simulink model "mariner_sim"  (R2018b)
settings: Solver=ode1  StartTime=0.0  StopTime=600  FixedStep=0.1  RelTol=1e-3
libraries: neural x408, simulink x2
(part 12 of 22)

== system mariner_sim/Plant/NN Plant mariner (no delta_dot) pre and post processing/Layer 6/Delays 1 ==
  "p{6}" : Inport  PortDimensions=24
      mask Display: e = 0.06;c1 = [120 230 180]/255;c2 = ([120 230 180]+0)/(256+128);c3 = ([120 230 180]+128)/(256+128);patch([0 1 1 0],[0 0 1 1],c1);patch([0 1 1 1-e 1-e 0+e],[0 0 1 1-e 0+e 0+e],c2);patch([0 0 1 1-e 0+e 0+e],[0 1 1 1-e 1-e 0+e],c3);plot([0 1 1 0 0],[0 0 1 1 0]);
  mux : Mux  Inputs=1
      mask Display: e = 0.06;c1 = [120 150 230]/255;c2 = ([120 150 230]+0)/383;c3 = ([120 150 230]+128)/383;patch([0 1 1 0],[0 0 1 1],c1);patch([0 1 1 1-e 1-e 0+e],[0 0 1 1-e 0+e 0+e],c2);patch([0 0 1 1-e 0+e 0+e],[0 1 1 1-e 1-e 0+e],c3);plot([0 1 1 0 0],[0 0 1 1 0]);disp('Mux')
  "pd{6,5}" : Outport
      mask Display: e = 0.06;c1 = [120 230 180]/255;c2 = ([120 230 180]+0)/(256+128);c3 = ([120 230 180]+128)/(256+128);patch([0 1 1 0],[0 0 1 1],c1);patch([0 1 1 1-e 1-e 0+e],[0 0 1 1-e 0+e 0+e],c2);patch([0 0 1 1-e 0+e 0+e],[0 1 1 1-e 1-e 0+e],c3);plot([0 1 1 0 0],[0 0 1 1 0]);
  wires:
  mux/1 -> "pd{6,5}"/1
  "p{6}"/1 -> mux/1

== system mariner_sim/Plant/NN Plant mariner (no delta_dot) pre and post processing/Layer 6/LW{6,5} ==
  "ad{6,5}" : Inport  PortDimensions=24
      mask Display: e = 0.06;c1 = [120 230 180]/255;c2 = ([120 230 180]+0)/(256+128);c3 = ([120 230 180]+128)/(256+128);patch([0 1 1 0],[0 0 1 1],c1);patch([0 1 1 1-e 1-e 0+e],[0 0 1 1-e 0+e 0+e],c2);patch([0 0 1 1-e 0+e 0+e],[0 1 1 1-e 1-e 0+e],c3);plot([0 1 1 0 0],[0 0 1 1 0]);
  "IW{6,5}(1,:)'" : Constant  Value=[-0.1984734159113137608176913317947764880955219268798828125;0.341861037683038826440196089606615714728832244873046875;0.3514792256180998553105609971680678427219390869140625;0.0708036460294599045983687801708583720028400421142578125;-0.2060005329274126051330995323951356112957000732421875;-0.28458774915436857444461793420487083494663238525390625;0.34526917716851002193578779042582027614116668701171875;0.252498381251613224218743880555848591029644012451171875;0.382796941171386462254844218477956019341945648193359375;0.1069087646510679390221554285744787193834781646728515625;0.265337792837605002116418972946121357381343841552734375;-0.0036982135335794073284498839626621702336706221103668212890625;0.097003491573064704045492590012145228683948516845703125;0.337797072626230543423986318884999491274356842041015625;-0.2407305535513760974541952464278438128530979156494140625;0.032264868090931257682552057985958526842296123504638671875;-0.09944305951370562002278319368997472338378429412841796875;-0.0237766981619511319490101186602259986102581024169921875;-0.368802813456096723054855601731105707585811614990234375;-0.0342788950269383996261041147590731270611286163330078125;-0.3817990555449328748949255896150134503841400146484375;-0.337620208706587543456834055177750997245311737060546875;0.2156801313526628127714701577133382670581340789794921875;0.487288760457548264515281744024832732975482940673828125]
      mask Display: e = 0.06;c1 = [120 150 230]/255;c2 = ([120 150 230]+0)/383;c3 = ([120 150 230]+128)/383;patch([0 1 1 0],[0 0 1 1],c1);patch([0 1 1 1-e 1-e 0+e],[0 0 1 1-e 0+e 0+e],c2);patch([0 0 1 1-e 0+e 0+e],[0 1 1 1-e 1-e 0+e],c3);plot([0 1 1 0 0],[0 0 1 1 0]);disp('weights');
  "IW{6,5}(2,:)'" : Constant  Value=[-0.09751875485376855501318260621701483614742755889892578125;0.01035142127946475643085477713611908257007598876953125;-0.0633120424566557538081923439676756970584392547607421875;0.1178993640669732390069412986122188158333301544189453125;0.09018636110401789807156092138029634952545166015625;-0.2332660662459413725144941054168157279491424560546875;0.06980453513620508976256218147682375274598598480224609375;0.1317458131781703845053499435380217619240283966064453125;-0.1974794491107817184794015474835759960114955902099609375;0.045960960379689101695799280378196272067725658416748046875;-0.0286857227069632104987650933480836101807653903961181640625;0.031652413341904737931198354772277525626122951507568359375;-0.1798477845368142979953773874512990005314350128173828125;0.113930975779332255282128016915521584451198577880859375;-0.1329135904041280069609598513125092722475528717041015625;0.1710109273118207984243355213038739748299121856689453125;-0.395146018496356277172054660695721395313739776611328125;0.0157313605677542878158448047543060965836048126220703125;-0.2089047495222683681337372263442375697195529937744140625;-0.012458230094540577448380958003326668404042720794677734375;0.1814413847518826783389300771887064911425113677978515625;0.16440010903084878446378525040927343070507049560546875;-0.0299410897703677979231340344767886563204228878021240234375;-0.291647538202252476491338484265725128352642059326171875]
      mask Display: e = 0.06;c1 = [120 150 230]/255;c2 = ([120 150 230]+0)/383;c3 = ([120 150 230]+128)/383;patch([0 1 1 0],[0 0 1 1],c1);patch([0 1 1 1-e 1-e 0+e],[0 0 1 1-e 0+e 0+e],c2);patch([0 0 1 1-e 0+e 0+e],[0 1 1 1-e 1-e 0+e],c3);plot([0 1 1 0 0],[0 0 1 1 0]);disp('weights');
  "IW{6,5}(3,:)'" : Constant  Value=[0.107561595046206937009714010855532251298427581787109375;0.11473176770232372534419340581735013984143733978271484375;0.09835083216250127546853576632202020846307277679443359375;-0.1101936730172489442569627726697945035994052886962890625;0.01956165002644803807552165153538226149976253509521484375;-0.00138938835503763674118771209720080150873400270938873291015625;0.229539681556379993043748299896833486855030059814453125;-0.02781216225646444828445424946039565838873386383056640625;-0.066868172082727606042595880353474058210849761962890625;-0.06345845663674787306973712475155480206012725830078125;-0.1061321176180718139914205266904900781810283660888671875;0.166181117806918077217659401867422275245189666748046875;0.049588349948201472516817744917716481722891330718994140625;0.038948608670263007436318503096117638051509857177734375;0.013791532259307952290594556643554824404418468475341796875;0.09946765208005929614909490510399336926639080047607421875;-0.11249367046046228335587358060365659184753894805908203125;-0.012219618567312066914620771740374038927257061004638671875;-0.16240728937219872651809282615431584417819976806640625;0.023389458205694983738975878395649488084018230438232421875;0.26389662063826035964808625067234970629215240478515625;0.159727556975424678231689767926582135260105133056640625;0.0754751463558475388371249437113874591886997222900390625;-0.17697164411906440850685839905054308474063873291015625]
      mask Display: e = 0.06;c1 = [120 150 230]/255;c2 = ([120 150 230]+0)/383;c3 = ([120 150 230]+128)/383;patch([0 1 1 0],[0 0 1 1],c1);patch([0 1 1 1-e 1-e 0+e],[0 0 1 1-e 0+e 0+e],c2);patch([0 0 1 1-e 0+e 0+e],[0 1 1 1-e 1-e 0+e],c3);plot([0 1 1 0 0],[0 0 1 1 0]);disp('weights');
  "IW{6,5}(4,:)'" : Constant  Value=[-0.024147515529926721900011443722178228199481964111328125;-0.115126686689287882625620795806753449141979217529296875;-0.13186707320813206845144804901792667806148529052734375;-0.045328318661101707487404155472177080810070037841796875;-0.2033729362155631548159107069295714609324932098388671875;0.07246896249946392642993231447690050117671489715576171875;-0.2179812681494835702178392011774121783673763275146484375;0.297405231087761456887363920031930319964885711669921875;0.032114410553897569655656951681521604768931865692138671875;0.04623473238628690584750557945881155319511890411376953125;-0.03509861948767252493031065796458278782665729522705078125;0.364105084360460573567053188526188023388385772705078125;-0.148060441730926084513697560396394692361354827880859375;0.3020276997199451418651960921124555170536041259765625;-0.1543730986813571515181564564045402221381664276123046875;0.10453222125549561927204678113412228412926197052001953125;0.0682407958586081220264674129794002510607242584228515625;0.03498961749381442054573909672399167902767658233642578125;-0.07624817135712991245100056403316557407379150390625;-0.010644929451439501255638475640807882882654666900634765625;-0.132186238467594530110460482319467701017856597900390625;0.320961225121417170758064685287536121904850006103515625;0.287195938470433009825910630752332508563995361328125;-0.112442449440882941136266026660450734198093414306640625]
      mask Display: e = 0.06;c1 = [120 150 230]/255;c2 = ([120 150 230]+0)/383;c3 = ([120 150 230]+128)/383;patch([0 1 1 0],[0 0 1 1],c1);patch([0 1 1 1-e 1-e 0+e],[0 0 1 1-e 0+e 0+e],c2);patch([0 0 1 1-e 0+e 0+e],[0 1 1 1-e 1-e 0+e],c3);plot([0 1 1 0 0],[0 0 1 1 0]);disp('weights');
  "IW{6,5}(5,:)'" : Constant  Value=[0.0265249665311167066861219865359089453704655170440673828125;-0.06515276408474486580235662813720409758388996124267578125;0.11698791214771177282560898902374901808798313140869140625;0.058168059701191376920093034641467966139316558837890625;0.033920652373470742968475377665527048520743846893310546875;-0.09949568443026289565889186405911459587514400482177734375;0.06389822026648651898117492464734823442995548248291015625;-0.007795113443349485811417753922114570741541683673858642578125;0.1501300297768707603385252014049910940229892730712890625;0.07298433793207532993552177913443301804363727569580078125;-0.045143535446797673771346381954572279937565326690673828125;0.013778305668310057707781624003473552875220775604248046875;-0.06351331399283564882463082312824553810060024261474609375;0.1773286164884585180967491169212735258042812347412109375;0.124255763394060136928231941055855713784694671630859375;0.0106476607074032399158358686008796212263405323028564453125;-0.10051592027657681172048143025676836259663105010986328125;0.040941784790665514126573043540702201426029205322265625;0.2495698746379401422590404990842216648161411285400390625;-0.057979253144741782488580383869702927768230438232421875;0.1432954740414220384803201113754766993224620819091796875;-0.12450573687530662458922137147965258918702602386474609375;0.0273682257852485462390479398209208738990128040313720703125;-0.0272394570136111520419763820655134622938930988311767578125]
      mask Display: e = 0.06;c1 = [120 150 230]/255;c2 = ([120 150 230]+0)/383;c3 = ([120 150 230]+128)/383;patch([0 1 1 0],[0 0 1 1],c1);patch([0 1 1 1-e 1-e 0+e],[0 0 1 1-e 0+e 0+e],c2);patch([0 0 1 1-e 0+e 0+e],[0 1 1 1-e 1-e 0+e],c3);plot([0 1 1 0 0],[0 0 1 1 0]);disp('weights');
  "IW{6,5}(6,:)'" : Constant  Value=[-0.2004844681319393473462042720711906440556049346923828125;0.128833455962125864591172330619883723556995391845703125;0.098423568038649877909307406298466958105564117431640625;0.144999619851042316209799309945083223283290863037109375;-0.132357170363239740051852777469321154057979583740234375;0.11375979409283366872163156813257955946028232574462890625;0.06915188401280171481833036750686005689203739166259765625;0.022246094065410081108691286999601288698613643646240234375;-0.11652469676553868505042288461481803096830844879150390625;0.05101664210318289371937083842567517422139644622802734375;-0.05340684599345039973439241975938784889876842498779296875;-0.07022774922811247932941114413551986217498779296875;-0.06459404659984717411713717183374683372676372528076171875;-0.09188557076911878229719121691232430748641490936279296875;-0.0280421329569854015095753396735744900070130825042724609375;-0.131619071904788553784015903147519566118717193603515625;-0.0087761563220312942268375167031990713439881801605224609375;-0.1562829536434182375881363213920849375426769256591796875;0.058614224683764086509807356151213753037154674530029296875;-0.04989826144070728941581904791746637783944606781005859375;-0.06141680902619907345130201292704441584646701812744140625;-0.0230427291839343344193036244860195438377559185028076171875;0.1430616608072586004585247110298951156437397003173828125;-0.10004233012849218786843863426838652230799198150634765625]
      mask Display: e = 0.06;c1 = [120 150 230]/255;c2 = ([120 150 230]+0)/383;c3 = ([120 150 230]+128)/383;patch([0 1 1 0],[0 0 1 1],c1);patch([0 1 1 1-e 1-e 0+e],[0 0 1 1-e 0+e 0+e],c2);patch([0 0 1 1-e 0+e 0+e],[0 1 1 1-e 1-e 0+e],c3);plot([0 1 1 0 0],[0 0 1 1 0]);disp('weights');
  Mux : Mux  Inputs=6
      mask Display: e = 0.06;c1 = [120 150 230]/255;c2 = ([120 150 230]+0)/383;c3 = ([120 150 230]+128)/383;patch([0 1 1 0],[0 0 1 1],c1);patch([0 1 1 1-e 1-e 0+e],[0 0 1 1-e 0+e 0+e],c2);patch([0 0 1 1-e 0+e 0+e],[0 1 1 1-e 1-e 0+e],c3);plot([0 1 1 0 0],[0 0 1 1 0]);disp('Mux');
  dotprod{1..6} (6 alike) : neural/Weight Functions/dotprod
  "lz{6,5}" : Outport
      mask Display: e = 0.06;c1 = [120 230 180]/255;c2 = ([120 230 180]+0)/(256+128);c3 = ([120 230 180]+128)/(256+128);patch([0 1 1 0],[0 0 1 1],c1);patch([0 1 1 1-e 1-e 0+e],[0 0 1 1-e 0+e 0+e],c2);patch([0 0 1 1-e 0+e 0+e],[0 1 1 1-e 1-e 0+e],c3);plot([0 1 1 0 0],[0 0 1 1 0]);
  wires:
  Mux/1 -> "lz{6,5}"/1
  dotprod6/1 -> Mux/6
  "IW{6,5}(6,:)'"/1 -> dotprod6/1
  dotprod5/1 -> Mux/5
  "IW{6,5}(5,:)'"/1 -> dotprod5/1
  dotprod4/1 -> Mux/4
  "IW{6,5}(4,:)'"/1 -> dotprod4/1
  dotprod3/1 -> Mux/3
  "IW{6,5}(3,:)'"/1 -> dotprod3/1
  dotprod2/1 -> Mux/2
  "IW{6,5}(2,:)'"/1 -> dotprod2/1
  dotprod1/1 -> Mux/1
  "ad{6,5}"/1 -> dotprod6/2, dotprod5/2, dotprod4/2, dotprod3/2, dotprod2/2, dotprod1/2
  "IW{6,5}(1,:)'"/1 -> dotprod1/1

== system mariner_sim/Plant/NN plant mariner (No delta_dot)/Layer 1/Delays 1 ==
  "p{1}" : Inport  PortDimensions=8
      mask Display: e = 0.06;c1 = [120 230 180]/255;c2 = ([120 230 180]+0)/(256+128);c3 = ([120 230 180]+128)/(256+128);patch([0 1 1 0],[0 0 1 1],c1);patch([0 1 1 1-e 1-e 0+e],[0 0 1 1-e 0+e 0+e],c2);patch([0 0 1 1-e 0+e 0+e],[0 1 1 1-e 1-e 0+e],c3);plot([0 1 1 0 0],[0 0 1 1 0]);
  mux : Mux  Inputs=1
      mask Display: e = 0.06;c1 = [120 150 230]/255;c2 = ([120 150 230]+0)/383;c3 = ([120 150 230]+128)/383;patch([0 1 1 0],[0 0 1 1],c1);patch([0 1 1 1-e 1-e 0+e],[0 0 1 1-e 0+e 0+e],c2);patch([0 0 1 1-e 0+e 0+e],[0 1 1 1-e 1-e 0+e],c3);plot([0 1 1 0 0],[0 0 1 1 0]);disp('Mux')
  "pd{1,1}" : Outport
      mask Display: e = 0.06;c1 = [120 230 180]/255;c2 = ([120 230 180]+0)/(256+128);c3 = ([120 230 180]+128)/(256+128);patch([0 1 1 0],[0 0 1 1],c1);patch([0 1 1 1-e 1-e 0+e],[0 0 1 1-e 0+e 0+e],c2);patch([0 0 1 1-e 0+e 0+e],[0 1 1 1-e 1-e 0+e],c3);plot([0 1 1 0 0],[0 0 1 1 0]);
  wires:
  mux/1 -> "pd{1,1}"/1
  "p{1}"/1 -> mux/1

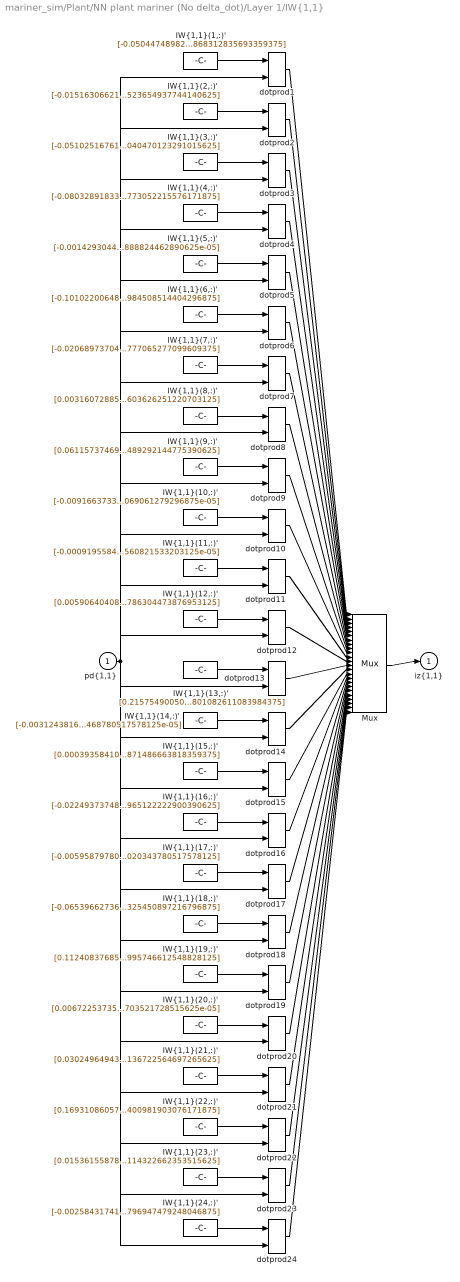
== system mariner_sim/Plant/NN plant mariner (No delta_dot)/Layer 1/IW{1,1} ==
  "pd{1,1}" : Inport  PortDimensions=8
      mask Display: e = 0.06;c1 = [120 230 180]/255;c2 = ([120 230 180]+0)/(256+128);c3 = ([120 230 180]+128)/(256+128);patch([0 1 1 0],[0 0 1 1],c1);patch([0 1 1 1-e 1-e 0+e],[0 0 1 1-e 0+e 0+e],c2);patch([0 0 1 1-e 0+e 0+e],[0 1 1 1-e 1-e 0+e],c3);plot([0 1 1 0 0],[0 0 1 1 0]);
  "IW{1,1}(1,:)'" : Constant  Value=[-0.050447489823092876715104893037278088741004467010498046875;-0.1453020904126429702074574379366822540760040283203125;0.1360442313365746447306747768379864282906055450439453125;0.083616133415922389016117222126922570168972015380859375;0.1859380844177798974836690604206523858010768890380859375;-0.0941200190030648531358536956759053282439708709716796875;-0.09836132576834526186626561639059218578040599822998046875;-0.0022978521690476898763078050791364148608408868312835693359375]
      mask Display: e = 0.06;c1 = [120 150 230]/255;c2 = ([120 150 230]+0)/383;c3 = ([120 150 230]+128)/383;patch([0 1 1 0],[0 0 1 1],c1);patch([0 1 1 1-e 1-e 0+e],[0 0 1 1-e 0+e 0+e],c2);patch([0 0 1 1-e 0+e 0+e],[0 1 1 1-e 1-e 0+e],c3);plot([0 1 1 0 0],[0 0 1 1 0]);disp('Weights');
  "IW{1,1}(10,:)'" : Constant  Value=[-0.00916637331366429268519890882771505857817828655242919921875;-0.0266038197254272502922933796298821107484400272369384765625;0.0179380205035220043063848294195850030519068241119384765625;0.07356487590796183251296014304898562841117382049560546875;0.073478906888268358255089651720481924712657928466796875;-0.0279816931304800974034119320776881068013608455657958984375;0.031718113041040503496947877692946349270641803741455078125;6.7575586318192662200858567000949506109463982284069061279296875e-05]
      mask Display: e = 0.06;c1 = [120 150 230]/255;c2 = ([120 150 230]+0)/383;c3 = ([120 150 230]+128)/383;patch([0 1 1 0],[0 0 1 1],c1);patch([0 1 1 1-e 1-e 0+e],[0 0 1 1-e 0+e 0+e],c2);patch([0 0 1 1-e 0+e 0+e],[0 1 1 1-e 1-e 0+e],c3);plot([0 1 1 0 0],[0 0 1 1 0]);disp('Weights');
  "IW{1,1}(11,:)'" : Constant  Value=[-0.0009195584270885333831591079700729096657596528530120849609375;-0.00444740981314047274797207620622430113144218921661376953125;0.00185387619551044395029004707708963906043209135532379150390625;-2.990664367495710310065719361727332170630688779056072235107421875e-05;0.00051533395249505546502344355275226917001418769359588623046875;-0.004831619154884273480143885848292484297417104244232177734375;-0.00394511335257156058042848911782130016945302486419677734375;5.913357744835549410951369697642121536773629486560821533203125e-05]
      mask Display: e = 0.06;c1 = [120 150 230]/255;c2 = ([120 150 230]+0)/383;c3 = ([120 150 230]+128)/383;patch([0 1 1 0],[0 0 1 1],c1);patch([0 1 1 1-e 1-e 0+e],[0 0 1 1-e 0+e 0+e],c2);patch([0 0 1 1-e 0+e 0+e],[0 1 1 1-e 1-e 0+e],c3);plot([0 1 1 0 0],[0 0 1 1 0]);disp('Weights');
  "IW{1,1}(12,:)'" : Constant  Value=[0.00590640408656031325185242764064241782762110233306884765625;0.00946153844084494412280950115246014320291578769683837890625;0.045269779862591112695735517945649917237460613250732421875;-0.003115516324658056113161563871472026221454143524169921875;-0.0408351532164521469070450621074996888637542724609375;0.0401849319427296791662485020424355752766132354736328125;0.00154371223938102285211382280749603523872792720794677734375;-0.00080467620072569652663052597318937841919250786304473876953125]
      mask Display: e = 0.06;c1 = [120 150 230]/255;c2 = ([120 150 230]+0)/383;c3 = ([120 150 230]+128)/383;patch([0 1 1 0],[0 0 1 1],c1);patch([0 1 1 1-e 1-e 0+e],[0 0 1 1-e 0+e 0+e],c2);patch([0 0 1 1-e 0+e 0+e],[0 1 1 1-e 1-e 0+e],c3);plot([0 1 1 0 0],[0 0 1 1 0]);disp('Weights');
  "IW{1,1}(13,:)'" : Constant  Value=[0.2157549005085194482322918929639854468405246734619140625;-0.21489809351830990724607772790477611124515533447265625;0.0288618450207983497091124291955566150136291980743408203125;-0.237729440761487886835112703920458443462848663330078125;-0.1626972710404361033287301552263670600950717926025390625;0.1747282626319985598950523808525758795440196990966796875;-0.0890875473259058192621040461744996719062328338623046875;-0.002758099109225537436118624867731341510079801082611083984375]
      mask Display: e = 0.06;c1 = [120 150 230]/255;c2 = ([120 150 230]+0)/383;c3 = ([120 150 230]+128)/383;patch([0 1 1 0],[0 0 1 1],c1);patch([0 1 1 1-e 1-e 0+e],[0 0 1 1-e 0+e 0+e],c2);patch([0 0 1 1-e 0+e 0+e],[0 1 1 1-e 1-e 0+e],c3);plot([0 1 1 0 0],[0 0 1 1 0]);disp('Weights');
  "IW{1,1}(14,:)'" : Constant  Value=[-0.0031243816162635413592740807331438190885819494724273681640625;-0.000928296421632138495268204980703785622608847916126251220703125;0.015765539928008949488447143494340707547962665557861328125;0.048519301693036365197286841066670604050159454345703125;0.06761290639592125450985093948474968783557415008544921875;-0.04476563135199958243237716715157148428261280059814453125;0.03100967803026542790600927901323302648961544036865234375;-9.452913233270264612047306673758839679067023098468780517578125e-05]
      mask Display: e = 0.06;c1 = [120 150 230]/255;c2 = ([120 150 230]+0)/383;c3 = ([120 150 230]+128)/383;patch([0 1 1 0],[0 0 1 1],c1);patch([0 1 1 1-e 1-e 0+e],[0 0 1 1-e 0+e 0+e],c2);patch([0 0 1 1-e 0+e 0+e],[0 1 1 1-e 1-e 0+e],c3);plot([0 1 1 0 0],[0 0 1 1 0]);disp('Weights');
  "IW{1,1}(15,:)'" : Constant  Value=[0.0003935841078905092890218020418302558027789928019046783447265625;-0.1219146255765612141264142564978101290762424468994140625;0.126057270212479644033720660445396788418292999267578125;0.26297717154439748110661412283661775290966033935546875;0.04385614172394687593214968046595458872616291046142578125;-0.1216715595383603132351169051617034710943698883056640625;-0.2243991548874049446471445889983442611992359161376953125;-0.00273468434944550663201479068220578483305871486663818359375]
      mask Display: e = 0.06;c1 = [120 150 230]/255;c2 = ([120 150 230]+0)/383;c3 = ([120 150 230]+128)/383;patch([0 1 1 0],[0 0 1 1],c1);patch([0 1 1 1-e 1-e 0+e],[0 0 1 1-e 0+e 0+e],c2);patch([0 0 1 1-e 0+e 0+e],[0 1 1 1-e 1-e 0+e],c3);plot([0 1 1 0 0],[0 0 1 1 0]);disp('Weights');
  "IW{1,1}(16,:)'" : Constant  Value=[-0.022493737485670149689465091569218202494084835052490234375;-0.02601958225636073762654376650971244089305400848388671875;0.0102396778713121604231783834393354482017457485198974609375;-0.00708757931484025986701436039538748445920646190643310546875;-0.00939306055311749099612228519617929123342037200927734375;-0.023126191692564530832942892857317929156124591827392578125;-0.011058591516381617581021856722145457752048969268798828125;0.0003539120631967357225901305017856657286756671965122222900390625]
      mask Display: e = 0.06;c1 = [120 150 230]/255;c2 = ([120 150 230]+0)/383;c3 = ([120 150 230]+128)/383;patch([0 1 1 0],[0 0 1 1],c1);patch([0 1 1 1-e 1-e 0+e],[0 0 1 1-e 0+e 0+e],c2);patch([0 0 1 1-e 0+e 0+e],[0 1 1 1-e 1-e 0+e],c3);plot([0 1 1 0 0],[0 0 1 1 0]);disp('Weights');
  "IW{1,1}(17,:)'" : Constant  Value=[-0.005958797805897233547389735264232513145543634891510009765625;-0.0093973397642727225786973832555304397828876972198486328125;-0.0012376240122008541448550555941210404853336513042449951171875;-0.00065132841794760822605458994161153896129690110683441162109375;-4.5122076628949407748996047740064341269317083060741424560546875e-05;-0.00805713876593570042794478780479039414785802364349365234375;-0.0102162154296771591488468544639545143581926822662353515625;0.0001810033460837132297804874525581908528693020343780517578125]
      mask Display: e = 0.06;c1 = [120 150 230]/255;c2 = ([120 150 230]+0)/383;c3 = ([120 150 230]+128)/383;patch([0 1 1 0],[0 0 1 1],c1);patch([0 1 1 1-e 1-e 0+e],[0 0 1 1-e 0+e 0+e],c2);patch([0 0 1 1-e 0+e 0+e],[0 1 1 1-e 1-e 0+e],c3);plot([0 1 1 0 0],[0 0 1 1 0]);disp('Weights');
  "IW{1,1}(18,:)'" : Constant  Value=[-0.0653966273670904818526850021953578107059001922607421875;-0.0035273106601568355276954402910405406146310269832611083984375;0.12142031588376388240302361509748152457177639007568359375;0.005048567160771975058375371503416317864321172237396240234375;-0.0230617190358675637484875409199958085082471370697021484375;0.12134561262626984701196164451175718568265438079833984375;-0.0821387603606360539032493761624209582805633544921875;-0.002553882405162404001242038020791369490325450897216796875]
      mask Display: e = 0.06;c1 = [120 150 230]/255;c2 = ([120 150 230]+0)/383;c3 = ([120 150 230]+128)/383;patch([0 1 1 0],[0 0 1 1],c1);patch([0 1 1 1-e 1-e 0+e],[0 0 1 1-e 0+e 0+e],c2);patch([0 0 1 1-e 0+e 0+e],[0 1 1 1-e 1-e 0+e],c3);plot([0 1 1 0 0],[0 0 1 1 0]);disp('Weights');
  "IW{1,1}(19,:)'" : Constant  Value=[0.112408376852322355876623305448447354137897491455078125;0.034998380185849616019755359275222872383892536163330078125;0.0209224337856189872286716280314067262224853038787841796875;0.0642909726389223334930278497267863713204860687255859375;0.10220346433478745551415300951703102327883243560791015625;-0.13228993400687627524092704334179870784282684326171875;0.004976469008829214994704681629400511155836284160614013671875;0.002518733874147201234894311028256197459995746612548828125]
      mask Display: e = 0.06;c1 = [120 150 230]/255;c2 = ([120 150 230]+0)/383;c3 = ([120 150 230]+128)/383;patch([0 1 1 0],[0 0 1 1],c1);patch([0 1 1 1-e 1-e 0+e],[0 0 1 1-e 0+e 0+e],c2);patch([0 0 1 1-e 0+e 0+e],[0 1 1 1-e 1-e 0+e],c3);plot([0 1 1 0 0],[0 0 1 1 0]);disp('Weights');
  "IW{1,1}(2,:)'" : Constant  Value=[-0.0151630662172396075970670636934301001019775867462158203125;-0.0173675527810003317574771841691472218371927738189697265625;0.006614564547864081218986331833775693667121231555938720703125;-0.004830036557984360330586515175355089013464748859405517578125;-0.006444823146448807639485867326811785460449755191802978515625;-0.01524339330352031569859594384297452052123844623565673828125;-0.007133693532216493944642099478414820623584091663360595703125;0.00024031351029684444088087291735433836947777308523654937744140625]
      mask Display: e = 0.06;c1 = [120 150 230]/255;c2 = ([120 150 230]+0)/383;c3 = ([120 150 230]+128)/383;patch([0 1 1 0],[0 0 1 1],c1);patch([0 1 1 1-e 1-e 0+e],[0 0 1 1-e 0+e 0+e],c2);patch([0 0 1 1-e 0+e 0+e],[0 1 1 1-e 1-e 0+e],c3);plot([0 1 1 0 0],[0 0 1 1 0]);disp('Weights');
  "IW{1,1}(20,:)'" : Constant  Value=[0.006722537357292009997655757302936763153411448001861572265625;0.0305504623949366636848079537003286532126367092132568359375;0.009990164157080559659274143768925569020211696624755859375;0.047101226865687857714437569711662945337593555450439453125;0.0905701070426076781938462545440415851771831512451171875;-0.051432578052114270861228106923590530641376972198486328125;0.061633932385347922622287342164781875908374786376953125;-4.2980567127764873779950660637183545986772514879703521728515625e-05]
      mask Display: e = 0.06;c1 = [120 150 230]/255;c2 = ([120 150 230]+0)/383;c3 = ([120 150 230]+128)/383;patch([0 1 1 0],[0 0 1 1],c1);patch([0 1 1 1-e 1-e 0+e],[0 0 1 1-e 0+e 0+e],c2);patch([0 0 1 1-e 0+e 0+e],[0 1 1 1-e 1-e 0+e],c3);plot([0 1 1 0 0],[0 0 1 1 0]);disp('Weights');
  "IW{1,1}(21,:)'" : Constant  Value=[0.03024964943486185831034163129515945911407470703125;0.003513838944816059621512049915281750145368278026580810546875;-0.03760875756503602451719103783034370280802249908447265625;0.033049628453540598471693812143712420947849750518798828125;0.0553194415863379196363069922881550155580043792724609375;-0.031522838468727686078718619455685256980359554290771484375;0.035462564650155244116991326563947950489819049835205078125;0.00205868014648965570734251429030337021686136722564697265625]
      mask Display: e = 0.06;c1 = [120 150 230]/255;c2 = ([120 150 230]+0)/383;c3 = ([120 150 230]+128)/383;patch([0 1 1 0],[0 0 1 1],c1);patch([0 1 1 1-e 1-e 0+e],[0 0 1 1-e 0+e 0+e],c2);patch([0 0 1 1-e 0+e 0+e],[0 1 1 1-e 1-e 0+e],c3);plot([0 1 1 0 0],[0 0 1 1 0]);disp('Weights');
  "IW{1,1}(22,:)'" : Constant  Value=[0.16931086057284649992737968204892240464687347412109375;0.1742700365394703465593551072743139229714870452880859375;-0.1293440059384691753763263477594591677188873291015625;0.1909964880266107056794311347402981482446193695068359375;-0.295806478986170129363841851954930461943149566650390625;0.558081381171123158679847620078362524509429931640625;-0.4608087767861663852642095662304200232028961181640625;0.000204232811886776821456990216319127284805290400981903076171875]
      mask Display: e = 0.06;c1 = [120 150 230]/255;c2 = ([120 150 230]+0)/383;c3 = ([120 150 230]+128)/383;patch([0 1 1 0],[0 0 1 1],c1);patch([0 1 1 1-e 1-e 0+e],[0 0 1 1-e 0+e 0+e],c2);patch([0 0 1 1-e 0+e 0+e],[0 1 1 1-e 1-e 0+e],c3);plot([0 1 1 0 0],[0 0 1 1 0]);disp('Weights');
  "IW{1,1}(23,:)'" : Constant  Value=[0.0153615587846137081895481202309383661486208438873291015625;-0.0216828073106015047077921309437442687340080738067626953125;0.05348196625824834515849914851060020737349987030029296875;-0.000874282336075373790740261625842322246171534061431884765625;-0.0202423698835987042610184971636044792830944061279296875;0.03694445685222873254627273809092002920806407928466796875;0.0047691140680123887685137873404528363607823848724365234375;-0.000711556687874899417879659413443960147560574114322662353515625]
      mask Display: e = 0.06;c1 = [120 150 230]/255;c2 = ([120 150 230]+0)/383;c3 = ([120 150 230]+128)/383;patch([0 1 1 0],[0 0 1 1],c1);patch([0 1 1 1-e 1-e 0+e],[0 0 1 1-e 0+e 0+e],c2);patch([0 0 1 1-e 0+e 0+e],[0 1 1 1-e 1-e 0+e],c3);plot([0 1 1 0 0],[0 0 1 1 0]);disp('Weights');
  "IW{1,1}(24,:)'" : Constant  Value=[-0.0025843174194612864892628412150088479393161833286285400390625;0.020602748877425726414802653607694082893431186676025390625;0.0149458391341018188847034053878815029747784137725830078125;0.02906000798233678017457037867643521167337894439697265625;0.045197937858079247075426820856591803021728992462158203125;-0.0200932242457597561025028909398315590806305408477783203125;0.0275179100843016798128015665270140743814408779144287109375;-0.000370446677698547314865062940469897512230090796947479248046875]
      mask Display: e = 0.06;c1 = [120 150 230]/255;c2 = ([120 150 230]+0)/383;c3 = ([120 150 230]+128)/383;patch([0 1 1 0],[0 0 1 1],c1);patch([0 1 1 1-e 1-e 0+e],[0 0 1 1-e 0+e 0+e],c2);patch([0 0 1 1-e 0+e 0+e],[0 1 1 1-e 1-e 0+e],c3);plot([0 1 1 0 0],[0 0 1 1 0]);disp('Weights');
  "IW{1,1}(3,:)'" : Constant  Value=[-0.051025167613189405246831853446565219201147556304931640625;-0.05810190480373868260333125590477720834314823150634765625;0.022165357503937277439121089628315530717372894287109375;-0.0180999625353478639511184411503563751466572284698486328125;-0.023099803347840099088106313729440444149076938629150390625;-0.04813471310499646549363461645043571479618549346923828125;-0.019984336874556647700718059468272258527576923370361328125;0.000803004852522657569004194133555074586183764040470123291015625]
      mask Display: e = 0.06;c1 = [120 150 230]/255;c2 = ([120 150 230]+0)/383;c3 = ([120 150 230]+128)/383;patch([0 1 1 0],[0 0 1 1],c1);patch([0 1 1 1-e 1-e 0+e],[0 0 1 1-e 0+e 0+e],c2);patch([0 0 1 1-e 0+e 0+e],[0 1 1 1-e 1-e 0+e],c3);plot([0 1 1 0 0],[0 0 1 1 0]);disp('Weights');
  "IW{1,1}(4,:)'" : Constant  Value=[-0.080328918333814114394186844947398640215396881103515625;-0.04037859471716932768803332010065787471830844879150390625;0.08500109009050739461432755206260480917990207672119140625;0.08778576971771183401482829822271014563739299774169921875;0.1594750323429694471855100346147082746028900146484375;-0.08008129311772292646676163485608412884175777435302734375;0.05174568048489840144110729625026579014956951141357421875;0.0002614332927247718196643588850491823905031196773052215576171875]
      mask Display: e = 0.06;c1 = [120 150 230]/255;c2 = ([120 150 230]+0)/383;c3 = ([120 150 230]+128)/383;patch([0 1 1 0],[0 0 1 1],c1);patch([0 1 1 1-e 1-e 0+e],[0 0 1 1-e 0+e 0+e],c2);patch([0 0 1 1-e 0+e 0+e],[0 1 1 1-e 1-e 0+e],c3);plot([0 1 1 0 0],[0 0 1 1 0]);disp('Weights');
  "IW{1,1}(5,:)'" : Constant  Value=[-0.0014293044614072832054763040332545642741024494171142578125;-0.00435308069703464577127061119199424865655601024627685546875;0.00150831464951281589252640724652110293391160666942596435546875;0.0022873501663876086124893571849270301754586398601531982421875;0.00136291520307263371199202328654109805938787758350372314453125;-0.003736825635841749086718532879558551940135657787322998046875;-0.0045455819879680996187243380290965433232486248016357421875;4.6299913404322865493646654844184240573667921125888824462890625e-05]
      mask Display: e = 0.06;c1 = [120 150 230]/255;c2 = ([120 150 230]+0)/383;c3 = ([120 150 230]+128)/383;patch([0 1 1 0],[0 0 1 1],c1);patch([0 1 1 1-e 1-e 0+e],[0 0 1 1-e 0+e 0+e],c2);patch([0 0 1 1-e 0+e 0+e],[0 1 1 1-e 1-e 0+e],c3);plot([0 1 1 0 0],[0 0 1 1 0]);disp('Weights');
  "IW{1,1}(6,:)'" : Constant  Value=[-0.10102200648479510436406059170622029341757297515869140625;0.025241785563793341096161526593277812935411930084228515625;0.04920978621778702988276421592672704719007015228271484375;-0.0165328354027705660966862666327870101667940616607666015625;-0.0219312143601313562502053144953606533817946910858154296875;0.0035411894430372793142469678429051782586611807346343994140625;0.033094292065775611499933717141175293363630771636962890625;-0.0011853844670704489876189580144227875280193984508514404296875]
      mask Display: e = 0.06;c1 = [120 150 230]/255;c2 = ([120 150 230]+0)/383;c3 = ([120 150 230]+128)/383;patch([0 1 1 0],[0 0 1 1],c1);patch([0 1 1 1-e 1-e 0+e],[0 0 1 1-e 0+e 0+e],c2);patch([0 0 1 1-e 0+e 0+e],[0 1 1 1-e 1-e 0+e],c3);plot([0 1 1 0 0],[0 0 1 1 0]);disp('Weights');
  "IW{1,1}(7,:)'" : Constant  Value=[-0.0206897370457268352239577069440201739780604839324951171875;-0.027644915611908439656563274411382735706865787506103515625;0.0164094506188974566252003484123633825220167636871337890625;-0.0097262934905449870137683632265179767273366451263427734375;-0.0143852525405528501589724754694543662481009960174560546875;-0.0166755870347807359788117054222311708144843578338623046875;0.000808590257662095417308389944111013392102904617786407470703125;0.0002902725318076354739903199853046089629060588777065277099609375]
      mask Display: e = 0.06;c1 = [120 150 230]/255;c2 = ([120 150 230]+0)/383;c3 = ([120 150 230]+128)/383;patch([0 1 1 0],[0 0 1 1],c1);patch([0 1 1 1-e 1-e 0+e],[0 0 1 1-e 0+e 0+e],c2);patch([0 0 1 1-e 0+e 0+e],[0 1 1 1-e 1-e 0+e],c3);plot([0 1 1 0 0],[0 0 1 1 0]);disp('Weights');
  "IW{1,1}(8,:)'" : Constant  Value=[0.003160728854689774484920672392718188348226249217987060546875;-0.013393341633646672905744168247110792435705661773681640625;0.038047579708717714497279160923426388762891292572021484375;0.0113964212934423887724211255090267513878643512725830078125;-0.00681852675149425928313728917373737203888595104217529296875;-0.0003156778285906476394680197916642327982117421925067901611328125;-0.0003260223775731108824572912485706410734564997255802154541015625;-0.000349180636884907917745490824046328270924277603626251220703125]
      mask Display: e = 0.06;c1 = [120 150 230]/255;c2 = ([120 150 230]+0)/383;c3 = ([120 150 230]+128)/383;patch([0 1 1 0],[0 0 1 1],c1);patch([0 1 1 1-e 1-e 0+e],[0 0 1 1-e 0+e 0+e],c2);patch([0 0 1 1-e 0+e 0+e],[0 1 1 1-e 1-e 0+e],c3);plot([0 1 1 0 0],[0 0 1 1 0]);disp('Weights');
  "IW{1,1}(9,:)'" : Constant  Value=[0.061157374690658905524998090186272747814655303955078125;0.04536019359910196946383820204573567025363445281982421875;0.05561722722852206757249149404742638580501079559326171875;-0.043541657094240508729665606324488180689513683319091796875;-0.0742405018223480095418409518970292992889881134033203125;0.122285780241033037452069720529834739863872528076171875;-0.0213096609083598363676426146184894605539739131927490234375;-0.0019626387438652207785561021324838293367065489292144775390625]
      mask Display: e = 0.06;c1 = [120 150 230]/255;c2 = ([120 150 230]+0)/383;c3 = ([120 150 230]+128)/383;patch([0 1 1 0],[0 0 1 1],c1);patch([0 1 1 1-e 1-e 0+e],[0 0 1 1-e 0+e 0+e],c2);patch([0 0 1 1-e 0+e 0+e],[0 1 1 1-e 1-e 0+e],c3);plot([0 1 1 0 0],[0 0 1 1 0]);disp('Weights');
  Mux : Mux  Inputs=24
      mask Display: e = 0.06;c1 = [120 150 230]/255;c2 = ([120 150 230]+0)/383;c3 = ([120 150 230]+128)/383;patch([0 1 1 0],[0 0 1 1],c1);patch([0 1 1 1-e 1-e 0+e],[0 0 1 1-e 0+e 0+e],c2);patch([0 0 1 1-e 0+e 0+e],[0 1 1 1-e 1-e 0+e],c3);plot([0 1 1 0 0],[0 0 1 1 0]);disp('Mux');
  dotprod{1..24} (24 alike) : neural/Weight Functions/dotprod
  "iz{1,1}" : Outport
      mask Display: e = 0.06;c1 = [120 230 180]/255;c2 = ([120 230 180]+0)/(256+128);c3 = ([120 230 180]+128)/(256+128);patch([0 1 1 0],[0 0 1 1],c1);patch([0 1 1 1-e 1-e 0+e],[0 0 1 1-e 0+e 0+e],c2);patch([0 0 1 1-e 0+e 0+e],[0 1 1 1-e 1-e 0+e],c3);plot([0 1 1 0 0],[0 0 1 1 0]);
  wires:
  Mux/1 -> "iz{1,1}"/1
  dotprod24/1 -> Mux/24
  "IW{1,1}(24,:)'"/1 -> dotprod24/1
  dotprod23/1 -> Mux/23
  "IW{1,1}(23,:)'"/1 -> dotprod23/1
  dotprod22/1 -> Mux/22
  "IW{1,1}(22,:)'"/1 -> dotprod22/1
  dotprod21/1 -> Mux/21
  "IW{1,1}(21,:)'"/1 -> dotprod21/1
  dotprod20/1 -> Mux/20
  "IW{1,1}(20,:)'"/1 -> dotprod20/1
  dotprod19/1 -> Mux/19
  "IW{1,1}(19,:)'"/1 -> dotprod19/1
  dotprod18/1 -> Mux/18
  "IW{1,1}(18,:)'"/1 -> dotprod18/1
  dotprod17/1 -> Mux/17
  "IW{1,1}(17,:)'"/1 -> dotprod17/1
  dotprod16/1 -> Mux/16
  "IW{1,1}(16,:)'"/1 -> dotprod16/1
  dotprod15/1 -> Mux/15
  "IW{1,1}(15,:)'"/1 -> dotprod15/1
  dotprod14/1 -> Mux/14
  "IW{1,1}(14,:)'"/1 -> dotprod14/1
  dotprod13/1 -> Mux/13
  "IW{1,1}(13,:)'"/1 -> dotprod13/1
  dotprod12/1 -> Mux/12
  "IW{1,1}(12,:)'"/1 -> dotprod12/1
  dotprod11/1 -> Mux/11
  "IW{1,1}(11,:)'"/1 -> dotprod11/1
  dotprod10/1 -> Mux/10
  "IW{1,1}(10,:)'"/1 -> dotprod10/1
  dotprod9/1 -> Mux/9
  "IW{1,1}(9,:)'"/1 -> dotprod9/1
  dotprod8/1 -> Mux/8
  "IW{1,1}(8,:)'"/1 -> dotprod8/1
  dotprod7/1 -> Mux/7
  "IW{1,1}(7,:)'"/1 -> dotprod7/1
  dotprod6/1 -> Mux/6
  "IW{1,1}(6,:)'"/1 -> dotprod6/1
  dotprod5/1 -> Mux/5
  "IW{1,1}(5,:)'"/1 -> dotprod5/1
  dotprod4/1 -> Mux/4
  "IW{1,1}(4,:)'"/1 -> dotprod4/1
  dotprod3/1 -> Mux/3
  "IW{1,1}(3,:)'"/1 -> dotprod3/1
  dotprod2/1 -> Mux/2
  "IW{1,1}(2,:)'"/1 -> dotprod2/1
  dotprod1/1 -> Mux/1
  "pd{1,1}"/1 -> dotprod24/2, dotprod23/2, dotprod22/2, dotprod21/2, dotprod20/2, dotprod19/2, dotprod18/2, dotprod17/2, dotprod16/2, dotprod15/2, dotprod14/2, dotprod13/2, dotprod12/2, dotprod11/2, dotprod10/2, dotprod9/2, dotprod8/2, dotprod7/2, dotprod6/2, dotprod5/2, dotprod4/2, dotprod3/2, dotprod2/2, dotprod1/2
  "IW{1,1}(1,:)'"/1 -> dotprod1/1

== system mariner_sim/Plant/NN plant mariner (No delta_dot)/Layer 2/Delays 1 ==
  "p{2}" : Inport  PortDimensions=24
      mask Display: e = 0.06;c1 = [120 230 180]/255;c2 = ([120 230 180]+0)/(256+128);c3 = ([120 230 180]+128)/(256+128);patch([0 1 1 0],[0 0 1 1],c1);patch([0 1 1 1-e 1-e 0+e],[0 0 1 1-e 0+e 0+e],c2);patch([0 0 1 1-e 0+e 0+e],[0 1 1 1-e 1-e 0+e],c3);plot([0 1 1 0 0],[0 0 1 1 0]);
  mux : Mux  Inputs=1
      mask Display: e = 0.06;c1 = [120 150 230]/255;c2 = ([120 150 230]+0)/383;c3 = ([120 150 230]+128)/383;patch([0 1 1 0],[0 0 1 1],c1);patch([0 1 1 1-e 1-e 0+e],[0 0 1 1-e 0+e 0+e],c2);patch([0 0 1 1-e 0+e 0+e],[0 1 1 1-e 1-e 0+e],c3);plot([0 1 1 0 0],[0 0 1 1 0]);disp('Mux')
  "pd{2,1}" : Outport
      mask Display: e = 0.06;c1 = [120 230 180]/255;c2 = ([120 230 180]+0)/(256+128);c3 = ([120 230 180]+128)/(256+128);patch([0 1 1 0],[0 0 1 1],c1);patch([0 1 1 1-e 1-e 0+e],[0 0 1 1-e 0+e 0+e],c2);patch([0 0 1 1-e 0+e 0+e],[0 1 1 1-e 1-e 0+e],c3);plot([0 1 1 0 0],[0 0 1 1 0]);
  wires:
  mux/1 -> "pd{2,1}"/1
  "p{2}"/1 -> mux/1
